simulink model "gm_DUALportRAMinterface_v3_vnl"  (R2024a)
settings: Solver=FixedStepDiscrete  StartTime=0.0  StopTime=0.1  RelTol=1e-3
undefined symbols (not defined in the file or in its folder): magnitude, Ts
libraries: hdlsllib x227, embmathops x6, simulink x2, hdlmdlgenlib x1, dsphdlxfrm2 x1
(part 6 of 6)

== stateflow chart gm_DUALportRAMinterface_v3_vnl/PL/integration_block1/GA_main/coefficent_array/Chart ==
  settings: executeAtInitialization=1
  state initial_sort
    during:
    index_increment = false;
    index_reset = true;
    swaps_increment = false;
    reset_swaps = true;
    sort_done = false;
  state round_increment
    entry:
    index_reset = true;
    reset_swaps = true;
  state not_perform_swap
    entry:
    commit_swap = 0;
  state start_round
    entry:
    reset_swaps = false;
    index_reset = false;
  state index_increment
    entry:
    index_increment = true;
    exit:
    index_increment = false;
  state perform_swap
    entry:
    commit_swap = index;
    swaps_increment = true;
    exit:
    commit_swap = 0;
    swaps_increment = false;
  state done_state
    entry:
    sort_done = true;
  (default) -> initial_sort
  done_state -> initial_sort
  initial_sort -> start_round : [start_sort]
  perform_swap -> round_increment [order 1] : [index == 3]
  not_perform_swap -> round_increment [order 3] : [index == 3]
  round_increment -> start_round
  start_round -> round_increment [order 2] : [index == 4]
  start_round -> not_perform_swap [order 1] : [swap_signal == false]
  not_perform_swap -> index_increment [order 1] : [index<3]
  not_perform_swap -> done_state [order 2] : [swaps_in == 0]
  start_round -> perform_swap [order 3] : [swap_signal == true]
  index_increment -> start_round
  perform_swap -> index_increment [order 2] : [index<3]
  data: index input; start_sort input; swaps_in input; index_increment output boolean; index_reset output boolean; sort_done output boolean; swap_signal input boolean; commit_swap output fixdt(0,4,0); swaps_increment output boolean; reset_swaps output boolean

== stateflow chart gm_DUALportRAMinterface_v3_vnl/PL/integration_block1/GA_main/coefficent_array1/Chart ==
  settings: executeAtInitialization=1
  state initial_sort
    during:
    index_increment = false;
    index_reset = true;
    swaps_increment = false;
    reset_swaps = true;
    sort_done = false;
  state round_increment
    entry:
    index_reset = true;
    reset_swaps = true;
  state not_perform_swap
    entry:
    commit_swap = 0;
  state start_round
    entry:
    reset_swaps = false;
    index_reset = false;
  state index_increment
    entry:
    index_increment = true;
    exit:
    index_increment = false;
  state perform_swap
    entry:
    commit_swap = index;
    swaps_increment = true;
    exit:
    commit_swap = 0;
    swaps_increment = false;
  state done_state
    entry:
    sort_done = true;
  (default) -> initial_sort
  done_state -> initial_sort
  initial_sort -> start_round : [start_sort]
  perform_swap -> round_increment [order 1] : [index == 3]
  not_perform_swap -> round_increment [order 3] : [index == 3]
  round_increment -> start_round
  start_round -> round_increment [order 2] : [index == 4]
  start_round -> not_perform_swap [order 1] : [swap_signal == false]
  not_perform_swap -> index_increment [order 1] : [index<3]
  not_perform_swap -> done_state [order 2] : [swaps_in == 0]
  start_round -> perform_swap [order 3] : [swap_signal == true]
  index_increment -> start_round
  perform_swap -> index_increment [order 2] : [index<3]
  data: index input; start_sort input; swaps_in input; index_increment output boolean; index_reset output boolean; sort_done output boolean; swap_signal input boolean; commit_swap output fixdt(0,4,0); swaps_increment output boolean; reset_swaps output boolean
